simulink model "ppo_position_attitude"  (R2025a)
settings: Solver=ode1  StartTime=0.0  StopTime=50  FixedStep=0.01  RelTol=1e-3
values from neighbouring files (symbols this model uses):
  control_noise = 0.045    [PPO_simulation.mat]    (also in TEST_POS_ATT_PPO.m)
  p_IC = IC(10)    [TEST_POS_ATT_PPO.m]
  phi_IC = IC(7)    [TEST_POS_ATT_PPO.m]
  psi_IC = IC(9)    [TEST_POS_ATT_PPO.m]
  q_IC = IC(11)    [TEST_POS_ATT_PPO.m]
  r_IC = IC(12)    [TEST_POS_ATT_PPO.m]
  state_noise = 0.045    [PPO_simulation.mat]    (also in TEST_POS_ATT_PPO.m)
  theta_IC = IC(8)    [TEST_POS_ATT_PPO.m]
  Ts_Sim = 0.01    [PPO_simulation.mat]    (also in TEST_POS_ATT_PPO.m)
  u_IC = IC(4)    [TEST_POS_ATT_PPO.m]
  v_IC = IC(5)    [TEST_POS_ATT_PPO.m]
  w_IC = IC(6)    [TEST_POS_ATT_PPO.m]
  x_IC = IC(1)    [TEST_POS_ATT_PPO.m]
  y_IC = IC(2)    [TEST_POS_ATT_PPO.m]
  z_IC = IC(3)    [TEST_POS_ATT_PPO.m]
undefined symbols (not defined in the file or in its folder): saturation_logic, wind_logic
libraries: rllib x2
settings Model: Creator=tn163528  LastModifiedBy=re606359

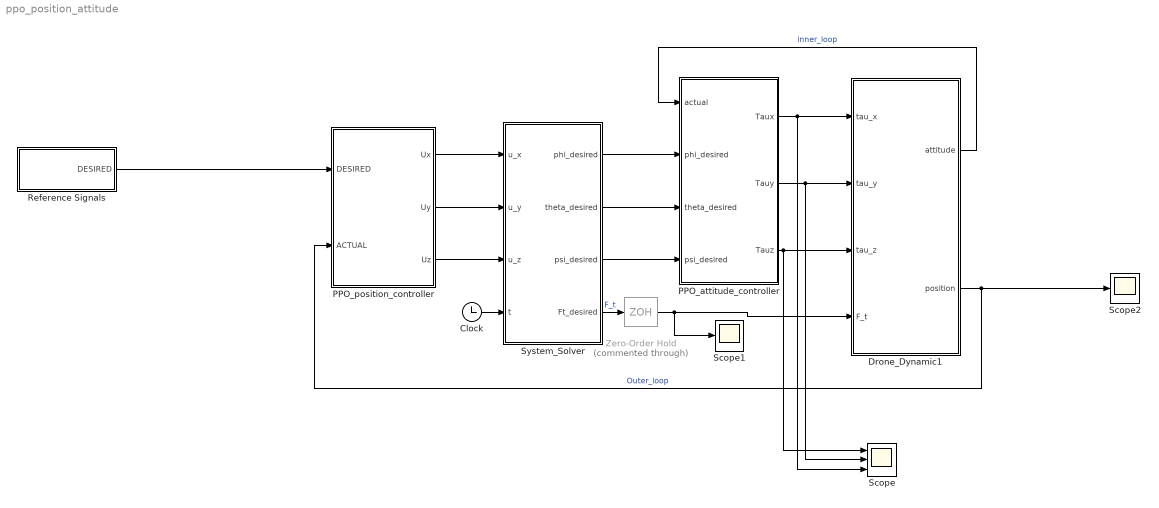
== system ppo_position_attitude ==
  Clock : Clock
  Drone_Dynamic1 : Subsystem
  PPO_attitude_controller : Subsystem
  PPO_position_controller : Subsystem
  Reference Signals : Subsystem
  Scope : Scope  NumInputPorts=3
      settings: ActiveDisplayYMinimum=-0.26589944162275436  ActiveDisplayYMaximum=0.67670267800432526  DataLoggingVariableName=ScopeData2
  Scope1 : Scope
      settings: ActiveDisplayYMinimum=72.877153012049746  ActiveDisplayYMaximum=83.875579825299113
  Scope2 : Scope
      settings: ActiveDisplayYMinimum=3.897727317905868  ActiveDisplayYMaximum=10.530186105155236  DataLoggingVariableName=ScopeData4
  System_Solver : MATLAB Function  TreatAsAtomicUnit=on
  Zero-Order Hold : ZeroOrderHold  Commented=through  SampleTime=.1
  wires:
  Reference Signals/1(DESIRED) -> PPO_position_controller/1(DESIRED)
  System_Solver/1(phi_desired) -> PPO_attitude_controller/2(phi_desired)
  Drone_Dynamic1/1(attitude) -> PPO_attitude_controller/1(actual)  "inner_loop"
  PPO_position_controller/1(Ux) -> System_Solver/1(u_x)
  PPO_position_controller/2(Uy) -> System_Solver/2(u_y)
  PPO_position_controller/3(Uz) -> System_Solver/3(u_z)
  System_Solver/2(theta_desired) -> PPO_attitude_controller/3(theta_desired)
  PPO_attitude_controller/1(Taux) -> Drone_Dynamic1/1(tau_x), Scope/3
  PPO_attitude_controller/2(Tauy) -> Drone_Dynamic1/2(tau_y), Scope/2
  PPO_attitude_controller/3(Tauz) -> Drone_Dynamic1/3(tau_z), Scope/1
  System_Solver/3(psi_desired) -> PPO_attitude_controller/4(psi_desired)
  Clock/1 -> System_Solver/4(t)
  Drone_Dynamic1/2(position) -> PPO_position_controller/2(ACTUAL), Scope2/1  "Outer_loop"
  System_Solver/4(Ft_desired) -> Zero-Order Hold/1  "F_t"
  Zero-Order Hold/1 -> Scope1/1, Drone_Dynamic1/4(F_t)

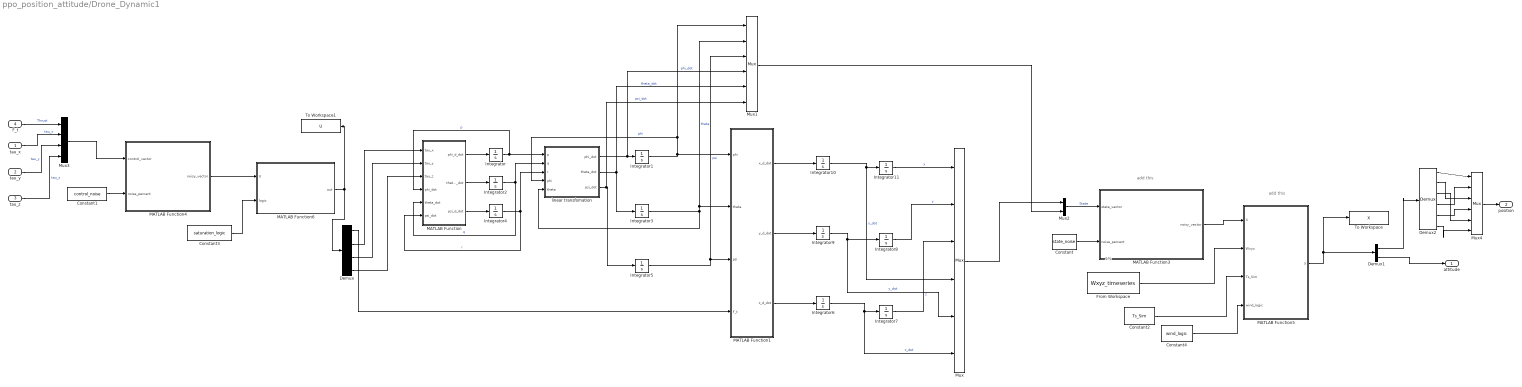
== system ppo_position_attitude/Drone_Dynamic1 ==
  note: add this
  note: add this
  note: 1%
  tau_x : Inport
  tau_y : Inport  Port=2
  tau_z : Inport  Port=3
  F_t : Inport  Port=4
  Constant : Constant  Value=state_noise  SampleTime=Ts_Sim
  Constant1 : Constant  Value=control_noise
  Constant2 : Constant  Value=Ts_Sim
  Constant3 : Constant  Value=saturation_logic  SampleTime=Ts_Sim
  Constant4 : Constant  Value=wind_logic
  Demux : Demux
  Demux1 : Demux  Outputs=2
  Demux2 : Demux  Outputs=6
  From Workspace : FromWorkspace  VariableName=Wxyz_timeseries  SampleTime=Ts_Sim
  Integrator : Integrator  InitialCondition=p_IC
  Integrator1 : Integrator  InitialCondition=phi_IC
  Integrator10 : Integrator  InitialCondition=u_IC
  Integrator11 : Integrator  InitialCondition=x_IC
  Integrator2 : Integrator  InitialCondition=q_IC
  Integrator3 : Integrator  InitialCondition=theta_IC
  Integrator4 : Integrator  InitialCondition=r_IC
  Integrator5 : Integrator  InitialCondition=psi_IC
  Integrator6 : Integrator  InitialCondition=w_IC
  Integrator7 : Integrator  InitialCondition=z_IC
  Integrator8 : Integrator  InitialCondition=y_IC
  Integrator9 : Integrator  InitialCondition=v_IC
  MATLAB Function : MATLAB Function  TreatAsAtomicUnit=on
  MATLAB Function1 : MATLAB Function  TreatAsAtomicUnit=on
  MATLAB Function3 : MATLAB Function  TreatAsAtomicUnit=on
  MATLAB Function4 : MATLAB Function  TreatAsAtomicUnit=on
  MATLAB Function5 : MATLAB Function  TreatAsAtomicUnit=on
  MATLAB Function6 : MATLAB Function  TreatAsAtomicUnit=on
  Mux : Mux  Inputs=6
  Mux1 : Mux  Inputs=6
  Mux2 : Mux  Inputs=2
  Mux3 : Mux
  Mux4 : Mux  Inputs=6
  To Workspace : ToWorkspace  VariableName=X  SampleTime=Ts_Sim
  To Workspace1 : ToWorkspace  VariableName=U  SampleTime=Ts_Sim
  linear transfomation : MATLAB Function  TreatAsAtomicUnit=on
  attitude : Outport
  position : Outport  Port=2
  wires:
  MATLAB Function1/1(x_d_dot) -> Integrator10/1
  MATLAB Function1/2(y_d_dot) -> Integrator9/1
  MATLAB Function1/3(z_d_dot) -> Integrator6/1
  Integrator1/1 -> Mux1/1, linear transfomation/4(phi), MATLAB Function1/1(phi)  "phi"
  Integrator3/1 -> Mux1/2, MATLAB Function1/2(theta), linear transfomation/5(theta)  "theta"
  Integrator5/1 -> Mux1/3, MATLAB Function1/3(psi)  "psi"
  Integrator10/1 -> Mux/4, Integrator11/1  "x_dot"
  Integrator9/1 -> Mux/5, Integrator8/1  "y_dot"
  Integrator6/1 -> Mux/6, Integrator7/1  "z_dot"
  Integrator2/1 -> MATLAB Function/5(theta_dot), linear transfomation/2(q)  "q"
  Integrator4/1 -> MATLAB Function/6(psi_dot), linear transfomation/3(r)  "r"
  Integrator/1 -> MATLAB Function/4(phi_dot), linear transfomation/1(p)  "p"
  MATLAB Function/3(psi_d_dot) -> Integrator4/1
  MATLAB Function/1(phi_d_dot) -> Integrator/1
  MATLAB Function/2(theta_d_dot) -> Integrator2/1
  linear transfomation/1(phi_dot) -> Mux1/4, Integrator1/1  "phi_dot"
  linear transfomation/2(theta_dot) -> Mux1/5, Integrator3/1  "theta_dot"
  linear transfomation/3(psi_dot) -> Mux1/6, Integrator5/1  "psi_dot"
  Integrator11/1 -> Mux/1  "x"
  Mux2/1 -> MATLAB Function3/1(state_vector)  "State"
  Constant/1 -> MATLAB Function3/2(noise_percent)
  MATLAB Function3/1(noisy_vector) -> MATLAB Function5/1("X ")
  Demux1/2 -> attitude/1
  From Workspace/1 -> MATLAB Function5/2(Wxyz)
  Constant2/1 -> MATLAB Function5/3(Ts_Sim)
  MATLAB Function5/1(X) -> To Workspace/1, Demux1/1
  Mux/1 -> Mux2/1
  Mux1/1 -> Mux2/2
  MATLAB Function4/1(noisy_vector) -> MATLAB Function6/1(U)
  Constant3/1 -> MATLAB Function6/2(logic)
  MATLAB Function6/1(out) -> Demux/1, To Workspace1/1
  Constant1/1 -> MATLAB Function4/2(noise_percent)
  F_t/1 -> Mux3/1  "Thrust"
  tau_x/1 -> Mux3/2  "tau_x"
  tau_y/1 -> Mux3/3  "tau_y"
  tau_z/1 -> Mux3/4  "tau_z"
  Mux3/1 -> MATLAB Function4/1(control_vector)
  Demux/1 -> MATLAB Function1/4(F_t)
  Demux/2 -> MATLAB Function/1(tau_x)
  Demux/3 -> MATLAB Function/2(tau_y)
  Demux/4 -> MATLAB Function/3(tau_z)
  Integrator8/1 -> Mux/2  "y"
  Integrator7/1 -> Mux/3  "z"
  Demux1/1 -> Demux2/1
  Demux2/1 -> Mux4/1
  Demux2/4 -> Mux4/2
  Demux2/2 -> Mux4/3
  Demux2/5 -> Mux4/4
  Demux2/3 -> Mux4/5
  Demux2/6 -> Mux4/6
  Mux4/1 -> position/1
  Constant4/1 -> MATLAB Function5/4(wind_logic)

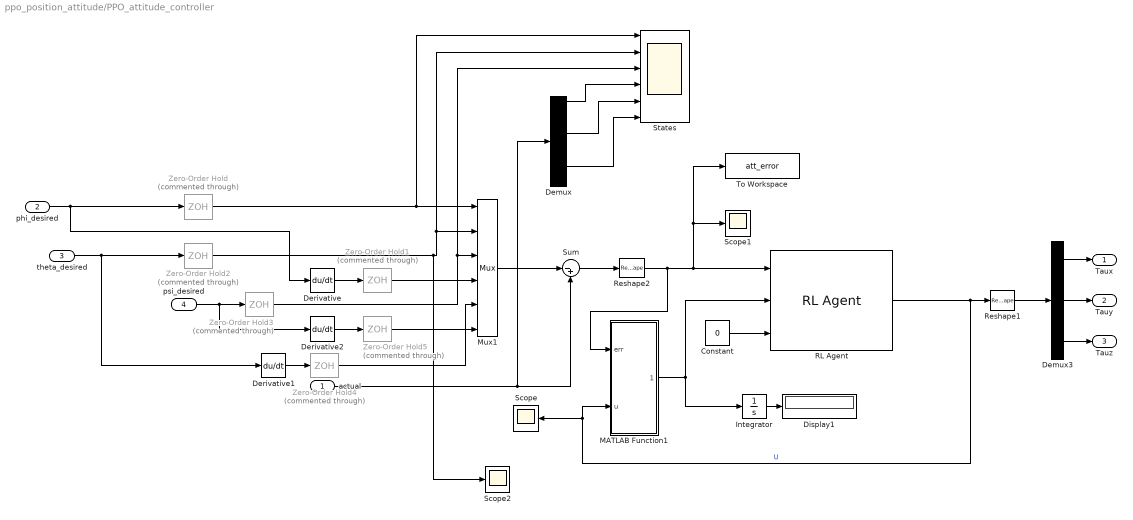
== system ppo_position_attitude/PPO_attitude_controller ==
  actual : Inport
  phi_desired : Inport  Port=2
  theta_desired : Inport  Port=3
  psi_desired : Inport  Port=4
  Constant : Constant  Value=0
  Demux : Demux  Outputs=6
  Demux3 : Demux  Outputs=3
  Derivative : Derivative
  Derivative1 : Derivative
  Derivative2 : Derivative
  Display1 : Display
  Integrator : Integrator
  MATLAB Function1 : MATLAB Function  TreatAsAtomicUnit=on
  Mux1 : Mux  Inputs=6
  RL Agent : rllib/RL Agent  Agent=agent1  ExternalActionAsInput=off  ProvideLastAction=off  ProvideCumRwd=off  TreatAsDirectFeedthrough=on  UseStrictObservationDataTypes=off
  Reshape1 : Reshape
  Reshape2 : Reshape  OutputDimensionality=Column vector (2-D)
  Scope : Scope
      settings: ActiveDisplayYMinimum=-0.20127  ActiveDisplayYMaximum=0.69251
  Scope1 : Scope
      settings: ActiveDisplayYMinimum=-1  ActiveDisplayYMaximum=1
  Scope2 : Scope
      settings: ActiveDisplayYMinimum=-0.040406254965963853  ActiveDisplayYMaximum=0.036209580605539526  DataLoggingVariableName=ScopeData3
  States : Scope  NumInputPorts=6
      settings: ActiveDisplayYMinimum=-0.042848507934818772  ActiveDisplayYMaximum=0.10576663107375736
  Sum : Sum  Inputs=|-+
  To Workspace : ToWorkspace  VariableName=att_error  SampleTime=Ts_Sim
  Zero-Order Hold{,1..5} (6 alike) : ZeroOrderHold  Commented=through  SampleTime=.1
  Taux : Outport
  Tauy : Outport  Port=2
  Tauz : Outport  Port=3
  wires:
  RL Agent/1 -> Scope/1, MATLAB Function1/2(u), Reshape1/1  "U"
  Constant/1 -> RL Agent/3
  Demux3/1 -> Taux/1
  Demux3/2 -> Tauy/1
  Demux3/3 -> Tauz/1
  phi_desired/1 -> Zero-Order Hold/1, Derivative/1
  theta_desired/1 -> Zero-Order Hold2/1, Derivative1/1
  psi_desired/1 -> Derivative2/1, Zero-Order Hold3/1
  Reshape1/1 -> Demux3/1
  Mux1/1 -> Sum/1
  actual/1 -> Demux/1, Sum/2
  Sum/1 -> Reshape2/1
  Reshape2/1 -> To Workspace/1, Scope1/1, RL Agent/1, MATLAB Function1/1(err)
  MATLAB Function1/1(reward) -> RL Agent/2, Integrator/1
  Integrator/1 -> Display1/1
  Demux/1 -> States/4
  Demux/3 -> States/5
  Demux/5 -> States/6
  Derivative/1 -> Zero-Order Hold1/1
  Derivative1/1 -> Zero-Order Hold4/1
  Derivative2/1 -> Zero-Order Hold5/1
  Zero-Order Hold/1 -> Mux1/1, States/1
  Zero-Order Hold1/1 -> Mux1/4
  Zero-Order Hold2/1 -> Scope2/1, Mux1/2, States/2
  Zero-Order Hold3/1 -> States/3, Mux1/3
  Zero-Order Hold4/1 -> Mux1/5
  Zero-Order Hold5/1 -> Mux1/6

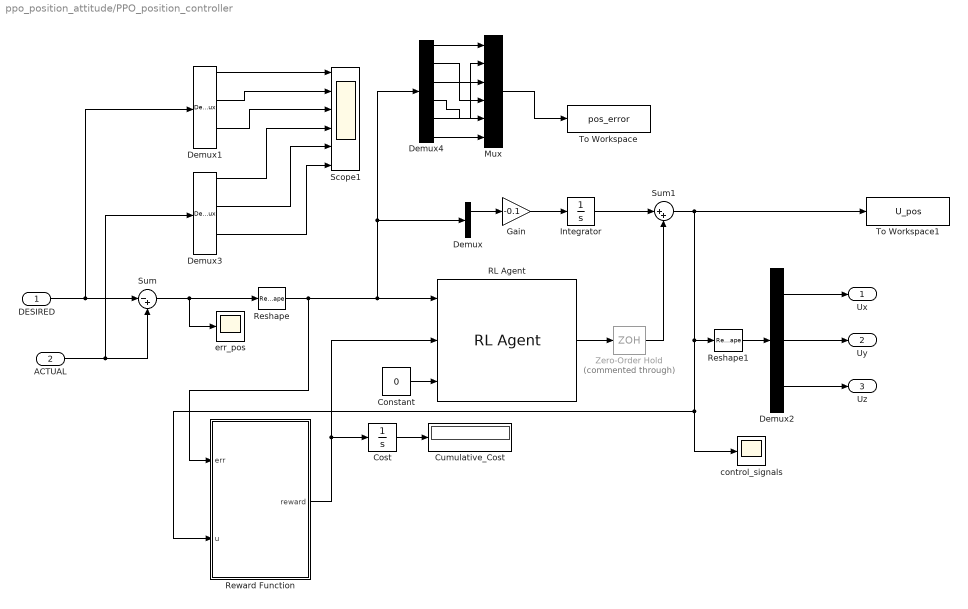
== system ppo_position_attitude/PPO_position_controller ==
  DESIRED : Inport
  ACTUAL : Inport  Port=2
  Constant : Constant  Value=0
  Cost : Integrator
  Cumulative_Cost : Display
  Demux : Demux  Outputs=2
  Demux1 : Demux  Outputs=6
  Demux2 : Demux  Outputs=3
  Demux3 : Demux  Outputs=6
  Demux4 : Demux  Outputs=6
  Gain : Gain  Gain=-0.1
  Integrator : Integrator
  Mux : Mux  Inputs=6
  RL Agent : rllib/RL Agent  Agent=agent  ExternalActionAsInput=off  ProvideLastAction=off  ProvideCumRwd=off  TreatAsDirectFeedthrough=on  UseStrictObservationDataTypes=off
  Reshape : Reshape  OutputDimensionality=Column vector (2-D)
  Reshape1 : Reshape
  Reward Function : MATLAB Function  TreatAsAtomicUnit=on
  Scope1 : Scope  NumInputPorts=6
      settings: ActiveDisplayYMinimum=-5.046617163465049  ActiveDisplayYMaximum=4.1195544711854284
  Sum : Sum  Inputs=|-+
  Sum1 : Sum  Inputs=|++
  To Workspace : ToWorkspace  VariableName=pos_error  SampleTime=Ts_Sim
  To Workspace1 : ToWorkspace  VariableName=U_pos  SampleTime=Ts_Sim
  Zero-Order Hold : ZeroOrderHold  Commented=through  SampleTime=.1
  control_signals : Scope
      settings: ActiveDisplayYMinimum=-0.47076  ActiveDisplayYMaximum=0.3367  DataLoggingVariableName=control_signal
  err_pos : Scope
      settings: ActiveDisplayYMinimum=-2.9375  ActiveDisplayYMaximum=1.4375  DataLoggingVariableName=control_signal1
  Ux : Outport
  Uy : Outport  Port=2
  Uz : Outport  Port=3
  wires:
  Demux2/1 -> Ux/1
  Demux2/2 -> Uy/1
  Demux2/3 -> Uz/1
  Reshape1/1 -> Demux2/1
  Reward Function/1(reward) -> Cost/1, RL Agent/2
  ACTUAL/1 -> Demux3/1, Sum/2
  DESIRED/1 -> Demux1/1, Sum/1
  Sum/1 -> Reshape/1, err_pos/1
  Reshape/1 -> Demux/1, Demux4/1, RL Agent/1, Reward Function/1(err)
  Cost/1 -> Cumulative_Cost/1
  Constant/1 -> RL Agent/3
  Demux1/1 -> Scope1/1
  Demux1/3 -> Scope1/2
  Demux1/5 -> Scope1/3
  Demux3/1 -> Scope1/4
  Demux3/3 -> Scope1/5
  Demux3/5 -> Scope1/6
  Gain/1 -> Integrator/1
  Demux/1 -> Gain/1
  Integrator/1 -> Sum1/1
  Sum1/1 -> To Workspace1/1, control_signals/1, Reward Function/2(u), Reshape1/1
  Demux4/1 -> Mux/1
  Mux/1 -> To Workspace/1
  Demux4/2 -> Mux/4
  Demux4/3 -> Mux/2
  Demux4/5 -> Mux/3
  Demux4/4 -> Mux/5
  Demux4/6 -> Mux/6
  RL Agent/1 -> Zero-Order Hold/1
  Zero-Order Hold/1 -> Sum1/2

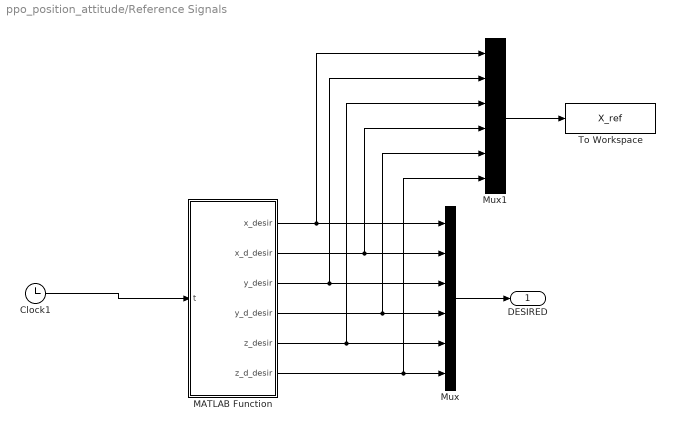
== system ppo_position_attitude/Reference Signals ==
  Clock1 : Clock
  MATLAB Function : MATLAB Function  TreatAsAtomicUnit=on
  Mux : Mux  Inputs=6
  Mux1 : Mux  Inputs=6
  To Workspace : ToWorkspace  VariableName=X_ref  SampleTime=Ts_Sim
  DESIRED : Outport
  wires:
  MATLAB Function/5(z_desir) -> Mux1/3, Mux/5
  MATLAB Function/1(x_desir) -> Mux1/1, Mux/1
  MATLAB Function/6(z_d_desir) -> Mux1/6, Mux/6
  MATLAB Function/2(x_d_desir) -> Mux1/4, Mux/2
  MATLAB Function/3(y_desir) -> Mux1/2, Mux/3
  Mux/1 -> DESIRED/1
  MATLAB Function/4(y_d_desir) -> Mux1/5, Mux/4
  Mux1/1 -> To Workspace/1
  Clock1/1 -> MATLAB Function/1(t)

== matlab function ppo_position_attitude/Drone_Dynamic1/linear transfomation ==
  data: p input; q input; r input; phi_dot output; phi input; theta input; theta_dot output; psi_dot output
function [phi_dot, theta_dot, psi_dot] = fcn(p,q,r, phi,theta)

    phi_dot   = p + (q*sin(phi)*tan(theta)) + (r*cos(phi)*tan(theta));
    theta_dot = (q*cos(phi)) - (r*sin(phi));
    psi_dot   = (q*sin(phi)/cos(theta)) + (r*cos(phi)/cos(theta));

end



    % if theta == deg2rad(90) || theta == deg2rad(-90)
    %    theta = sign(theta)*deg2rad(89.9); 
    % end

% 89.9 value is fixed. 
% if change to 89.99, phi_dot and psi_dot value will explode.

== matlab function ppo_position_attitude/Drone_Dynamic1/MATLAB Function4 ==
  settings: updateMethod=DISCRETE
  data: control_vector input; noisy_vector output; noise_percent input
function noisy_vector = add_control_noise(control_vector, noise_percent)

    L = 0.2;
    % drag = 0.02; % (drag coef)
    max_Ft = 2*9.81;
    Tmax = max_Ft/4;
    Max_torque = Tmax*L*2;
    actuator_uncert = [0.1*max_Ft, 0.01*Max_torque, 0.01*Max_torque, 0.02*Max_torque]';
    
    noise = (noise_percent) * actuator_uncert .* randn(size(control_vector)); % noise_percent 1 2 3 4 5
    noisy_vector = control_vector + noise;
    
end

== matlab function ppo_position_attitude/Drone_Dynamic1/MATLAB Function6 ==
  data: U input; out output; logic input
% saturation function
function out = saturate_controls(U, logic)

    if logic == 1

        ft = U(1);
        torques = [U(2); U(3); U(4)];
        m = 1;
        g = 9.81;
        L = 0.2;
        drag = 0.02; % (drag coef)
        max_Ft = 2*m*g;
        Tmin = 0;
        Tmax = max_Ft/4;
        max_torque = Tmax*L*2;
        max_yaw_torque = 0.7*max_torque;

        % saturate the torques to the max torque the drone can produce
        for p = 1:2 % sat the first 2
            if torques(p) > max_torque
                torques(p) = max_torque;
            elseif torques(p) < -max_torque
                torques(p) = -max_torque;
            end
        end
        if torques(3) > max_yaw_torque
            torques(3) = max_yaw_torque;
        elseif torques(3) < -max_yaw_torque
            torques(3) = -max_yaw_torque;
        end
        % solve for the thrust of each motor given those torques
        T1 = (ft - torques(1)/(2*L) - torques(2)/(2*L) + torques(3)/(4*drag)) / 4;
        T2 = (ft - torques(1)/(2*L) + torques(2)/(2*L) + torques(3)/(4*drag)) / 4;
        T3 = (ft + torques(1)/(2*L) - torques(2)/(2*L) - torques(3)/(4*drag)) / 4;
        T4 = (ft + torques(1)/(2*L) + torques(2)/(2*L) - torques(3)/(4*drag)) / 4;
        each_motor_thrust = [T1;T2;T3;T4];

        % saturate each motor thrust to its bounded values
        for j = 1:4
            if each_motor_thrust(j) > Tmax
                each_motor_thrust(j) = Tmax;
            elseif each_motor_thrust(j) < Tmin
                each_motor_thrust(j) = Tmin;
            end
        end

        ft = sum(each_motor_thrust);

        if ft>max_Ft
            ft = max_Ft;
        elseif ft<0
            ft = 0;
        end

        out = [ft; torques];

    else
    
        out = U;
    
    end


end

== matlab function ppo_position_attitude/PPO_position_controller/Reward Function ==
  data: err input; u input; reward output
function reward  = fcn(err, u)

    % reward = -0.1 * (err.' * Q_pos * err + u.' * R_pos * u);
    err1 = err(1); % x
    err2 = err(2); % x_dot
    err3 = err(3);
    err4 = err(4);
    err5 = err(5);
    err6 = err(6);

    ux = u(1);
    uy = u(2);
    uz = u(3);

    reward = -0.05*(1*abs(err1) + 0.1*abs(err2) + 1*abs(err3) + 0.1*abs(err4) + ...
                    1*abs(err5) + 0.1*abs(err6) + 0.1*abs(ux) + 0.1*abs(uy) + 0.1*abs(uz));

end

== matlab function ppo_position_attitude/System_Solver ==
  data: phi_desired output; theta_desired output; psi_desired output; u_x input; Ft_desired output; u_y input; u_z input; t input
function [phi_desired, theta_desired, psi_desired, Ft_desired] = fcn(u_x, u_y, u_z, t)
    
    m = 1;
    psi_desired = 0.09;
    u_z = 9.81-u_z;
    Ft_desired = m * sqrt(u_x^2 + u_y^2 + u_z^2);
    phi_desired = asin((u_y*m)/Ft_desired);
    theta_desired = asin((-u_x*m) / (Ft_desired*cos(phi_desired)));

    %% the method below should work identically, use either 
    % a = sin(psi_desired); %sin(0) = 0
    % b = cos(psi_desired); %cos(0) = 1
    % A = u_x/u_z;
    % B = u_y/u_z;
    % C = (a*A - b*B) / ( (a^2) + (b^2));
    % phi_desired = atan((B + b*C) / a);
    % theta_desired = atan(C * cos(phi_desired));
    %%
    phi_desired = phi_desired *(1-exp(-2*t));
    theta_desired = theta_desired * (1-exp(-2*t));
    if phi_desired > pi/6
        phi_desired = pi/6;
    elseif phi_desired < -pi/6
        phi_desired = -pi/6;
    end
    %%
    if theta_desired > pi/6
        theta_desired = pi/6;
    elseif theta_desired < -pi/6
        theta_desired = -pi/6;
    end
    % Ft_desired = (m / (cos(theta_desired) * cos(phi_desired))) * (-u_z);
end

== matlab function ppo_position_attitude/Drone_Dynamic1/MATLAB Function5 ==
  data: X input; Wxyz input; X output; Ts_Sim input; wind_logic input
function X = wind_f_m( X,Wxyz, Ts_Sim,  wind_logic)

    Cd = [.8; 0.8;1.2]; % Drag coefficient
    L = 0.2; % Half arm length (m)
    h = 0.05;
    A = [L*2*h, L*2*h, 2*L*L]; % Approximate frontal areas [x, y, z] in m^2
    r = [ L,  L, -L, -L;   % X positions of motors
          L, -L, -L,  L;   % Y positions of motors
          0,  0,  0,  0 ]; % Z positions (motors at same height)
    rho = 1.225; % Air density (kg/m^3)

    Ix = 0.3; Iy = 0.4; Iz = 0.5; m = 1;
    if wind_logic ==1
        R = eul2rotm_zyx( X(7), X(8), X(9) );
        Wxyz_body = R'*Wxyz;
        V_rel = X(4:6) - Wxyz_body;
        F_wind = -0.5 * rho * Cd .*diag(A) * (V_rel .* abs(V_rel)); % Compute wind forces
        
        F_wind_motors = repmat(F_wind, 1, 4) + 0.01*randn(3,4);
    
        M_wind_motors = cross(r, F_wind_motors, 1);
        M_wind = sum(M_wind_motors, 2);  
        
        accn_dist = F_wind/m;
        alpha_dist=    [M_wind(1)/Ix;
                        M_wind(2)/Iy;
                        M_wind(3)/Iz];
    
        X = X + Ts_Sim * [0;0;0;
                         accn_dist;
                         0;0;0;
                         alpha_dist];
    end
end

== matlab function ppo_position_attitude/Drone_Dynamic1/MATLAB Function3 ==
  settings: updateMethod=DISCRETE
  data: state_vector input; noisy_vector output; noise_percent input
function noisy_vector = add_state_noise(state_vector,noise_percent)

    sensor_uncert = [0.02, 0.02, 0.05, 0.05, 0.05, 0.05, 0.15, 0.15, 0.5, 0.005, 0.005, 0.005]';
  
    noise = (noise_percent) * sensor_uncert .* randn(size(state_vector)); % 0.01 usually add noise_percent 1 2 3 4 5
    noisy_vector = state_vector + noise;

end

== matlab function ppo_position_attitude/PPO_attitude_controller/MATLAB Function1 ==
  data: err input; reward output; u input
function reward = fcn(err,u)
    err1 = err(1); % phi
    err2 = err(2); % phi_dot
    err3 = err(3);
    err4 = err(4);
    err5 = err(5);
    err6 = err(6);

    ux = u(1);
    uy = u(2);
    uz = u(3);

    reward = -1*(1*abs(err1) + 0.1*abs(err2) + 1*abs(err3) + 0.1*abs(err4) + ...
                    1*abs(err5) + 0.1*abs(err6) + 0.1*abs(ux) + 0.1*abs(uy) + 0.01*abs(uz));

end

== matlab function ppo_position_attitude/Drone_Dynamic1/MATLAB Function ==
  data: tau_x input; tau_y input; tau_z input; phi_d_dot output; theta_d_dot output; psi_d_dot output; phi_dot input; theta_dot input; psi_dot input
function [phi_d_dot, theta_d_dot, psi_d_dot] = fcn(tau_x, tau_y, tau_z, phi_dot, theta_dot, psi_dot)
    I_x = 0.3; I_y = 0.4; I_z = 0.5;
    phi_d_dot = (((I_y - I_z)/I_x) * theta_dot * psi_dot) + (tau_x/I_x);
    theta_d_dot = (((I_z - I_x)/I_y) * phi_dot * psi_dot) + (tau_y/I_y);
    psi_d_dot = (((I_x - I_y)/I_z) * phi_dot * psi_dot) + (tau_z/I_z);
end

== matlab function ppo_position_attitude/Drone_Dynamic1/MATLAB Function1 ==
  data: phi input; x_d_dot output; theta input; psi input; F_t input; y_d_dot output; z_d_dot output
function [x_d_dot, y_d_dot, z_d_dot] = fcn(phi, theta, psi, F_t)
    m = 1; %1kg
    g = 9.81;
    x_d_dot= -(F_t/m) * (sin(phi)*sin(psi) + cos(phi)*cos(psi)*sin(theta));
    y_d_dot= -(F_t/m) * (cos(phi)*sin(psi)*sin(theta) - cos(psi)*sin(phi));
    z_d_dot= g-(F_t/m) * (cos(phi) * cos(theta));
end

== matlab function ppo_position_attitude/Reference Signals/MATLAB Function ==
  data: t input; x_desir output; x_d_desir output; y_desir output; y_d_desir output; z_desir output; z_d_desir output
function [x_desir, x_d_desir, y_desir, y_d_desir,...
    z_desir, z_d_desir] = trajectory_generator(t)
% trajectory_generator generates desired position and velocity.
    
    % x_desir = 10 * sin(0.25*t);
    % x_d_desir = 2.5 * cos(0.25*t);
    % y_desir = 70 * (1-exp(-0.01*t)) * cos(0.2*t);
    % y_d_desir = 70*(0.01*exp(-0.01*t))*cos(0.2*t) - 14*(1-exp(-0.01*t))*sin(0.2*t);
    
    %% helix
    % x_desir = (1-exp(-0.01*t))*9.81*cos(0.2*t);
    % x_d_desir = 9.81 * (0.01 * exp(-0.01 * t) * cos(0.2 * t) - 0.2 * (1 - exp(-0.01 * t)) * sin(0.2 * t));
    % y_desir = (1-exp(-0.01*t))*9.81*sin(0.2*t);
    % y_d_desir =  9.81 * (0.2 * (1 - exp(-0.01*t)) * cos(0.2*t) + 0.01 * exp(-0.01*t) * sin(0.2*t));
    % z_desir = -0.1*t;
    % z_d_desir = -0.1;

    %% crown path 
    x_desir = 9.81*cos(0.2*t);
    x_d_desir = -1.962*sin(0.2*t);

    y_desir = 9.81*sin(0.2*t);
    y_d_desir =  1.962*cos(0.2*t);
    
    z_desir = -4*cos(1*t)-9.81;
    z_d_desir = 4*sin(t);

    % x_desir = 0;
    % x_d_desir = 0;
    % y_desir = 0;
    % y_d_desir =  0;
    % z_desir = -0.1*t;
    % z_d_desir = -0.1;
end
